simulink model "phase3_bouc_wen"  (R2026a)
settings: Solver=VariableStepAuto
libraries: simulink x2
settings Model: Creator=User  LastModifiedBy=User

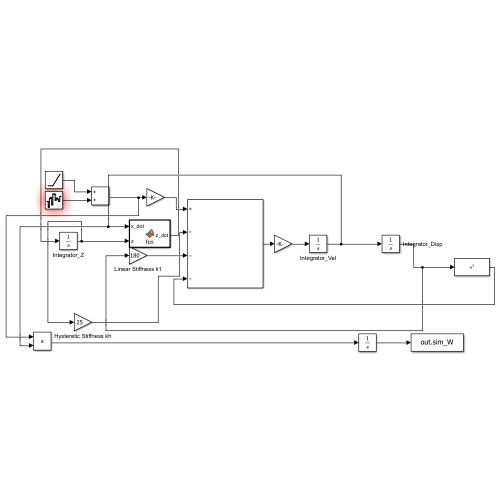
[thumbnail: Simulink's stored preview of the top-level diagram]
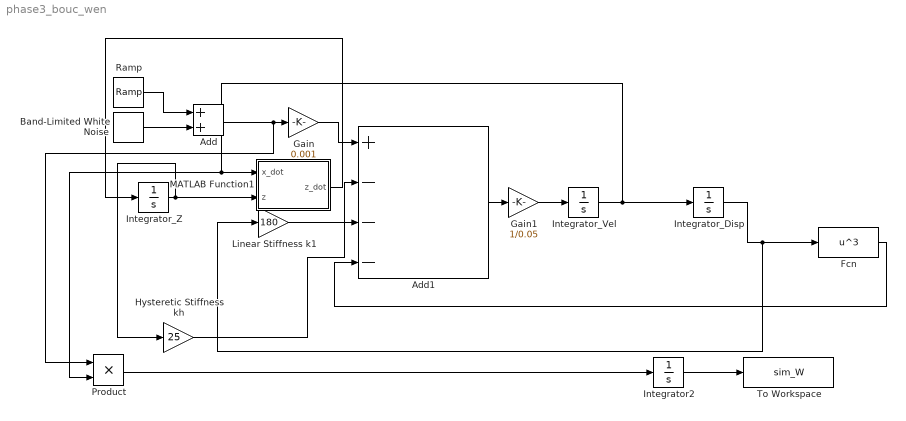
== system phase3_bouc_wen ==
  Add : Sum
  Add1 : Sum  Inputs=+---
  Band-Limited White Noise : simulink/Sources/Band-Limited White Noise  Cov=0.1  Ts=0.1  seed=noise_seed
  Fcn : Fcn  Expr=u^3
  Gain : Gain  Gain=0.001
  Gain1 : Gain  Gain=1/0.05
  Hysteretic Stiffness kh : Gain  Gain=25
  Integrator2 : Integrator
  Integrator_Disp : Integrator
  Integrator_Vel : Integrator
  Integrator_Z : Integrator
  Linear Stiffness k1 : Gain  Gain=180
  MATLAB Function1 : MATLAB Function  TreatAsAtomicUnit=on
  Product : Product
  Ramp : simulink/Sources/Ramp  slope=3000  start=0.1  InitialOutput=0
  To Workspace : ToWorkspace  VariableName=sim_W  SampleTime=-1
  wires:
  Integrator_Vel/1 -> Product/2, MATLAB Function1/1(x_dot), Integrator_Disp/1
  Band-Limited White Noise/1 -> Add/2
  Add/1 -> Product/1, Gain/1
  Gain/1 -> Add1/1
  Add1/1 -> Gain1/1
  Gain1/1 -> Integrator_Vel/1
  Linear Stiffness k1/1 -> Add1/3
  Integrator_Disp/1 -> Linear Stiffness k1/1, Fcn/1
  Fcn/1 -> Add1/4
  Product/1 -> Integrator2/1
  Integrator2/1 -> To Workspace/1
  Ramp/1 -> Add/1
  Integrator_Z/1 -> MATLAB Function1/2(z), Hysteretic Stiffness kh/1
  MATLAB Function1/1(z_dot) -> Integrator_Z/1
  Hysteretic Stiffness kh/1 -> Add1/2

== matlab function phase3_bouc_wen/MATLAB Function1 ==
  data: x_dot input; z_dot output; z input
function z_dot = fcn(x_dot, z)
% Bouc-Wen Hysteresis parameters for soft silicone (n=1)
A = 1.0;
beta = 1.5;
gamma = 0.5;

% The Bouc-Wen differential equation
z_dot = A * x_dot - beta * abs(x_dot) * z - gamma * x_dot * abs(z);
end
